simulink model "SISO_Timer"  (R2024a)
settings: Solver=VariableStepAuto  StartTime=0.0  StopTime=30  RelTol=1e-3
undefined symbols (not defined in the file or in its folder): BOOL, DINT, slplc
(part 2 of 3)

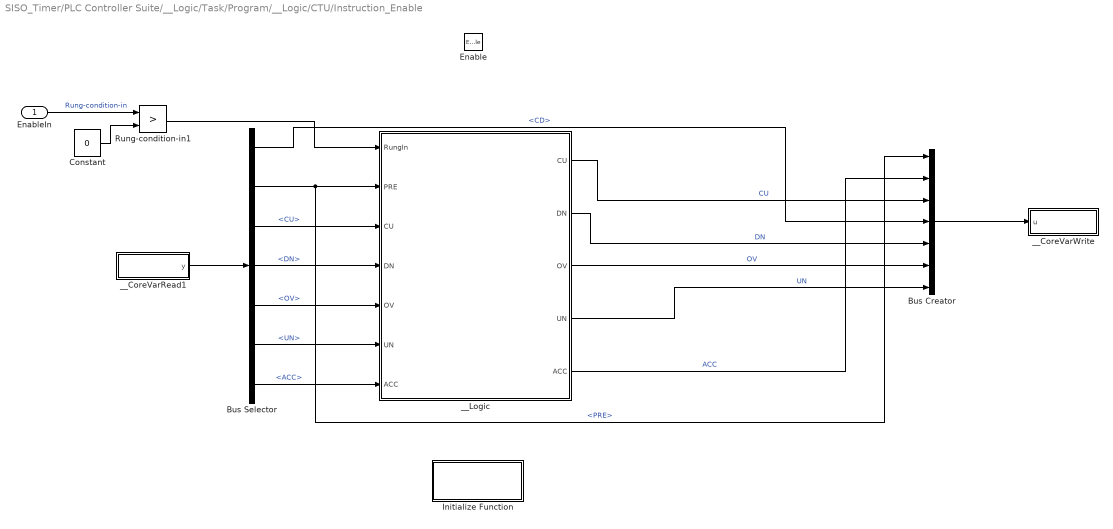
== system SISO_Timer/PLC Controller Suite/__Logic/Task/Program/__Logic/CTU/Instruction_Enable ==
  EnableIn : Inport
  Enable : EnablePort
  Bus Creator : BusCreator  Inputs=7  OutDataTypeStr=Bus: COUNTER  NonVirtualBus=on
  Bus Selector : BusSelector  OutputSignals=CD,PRE,CU,DN,OV,UN,ACC
  Constant : Constant  Value=0
  Initialize Function : Subsystem  TreatAsAtomicUnit=on
  Rung-condition-in1 : RelationalOperator  Operator=>  OutDataTypeStr=boolean  RndMeth=Simplest  InputSameDT=off
  __CoreVarRead1 : Subsystem  Tag=CoreVarReadBlock  DisableCoverage=on  TreatAsAtomicUnit=on  mask{PLCBlockType=CoreVarRead}
      mask init:
      | slplc.callbacks.initCoreVariable(gcb, 'read');
      mask Help: web([docroot '/plccoder/ref/__corevarread' '.html']);
      mask DialogControl PLCBlockTitle Prompt: Core Variable Read
  __CoreVarWrite : Subsystem  Tag=CoreVarWriteBlock  DisableCoverage=on  TreatAsAtomicUnit=on  mask{PLCBlockType=CoreVarWrite}
      mask init:
      | slplc.callbacks.initCoreVariable(gcb, 'write');
      mask Help: web([docroot '/plccoder/ref/__corevarwrite' '.html']);
      mask DialogControl PLCBlockTitle Prompt: Core Variable Write
  __Logic : MATLAB Function  Priority=12  DisableCoverage=on
  wires:
  Rung-condition-in1/1 -> __Logic/1(RungIn)
  Bus Selector/5 -> __Logic/5("OV ")  "<OV>"
  __Logic/4(UN) -> Bus Creator/7  "UN"
  Bus Selector/7 -> __Logic/7("ACC ")  "<ACC>"
  Bus Creator/1 -> __CoreVarWrite/1(u)
  __Logic/2(DN) -> Bus Creator/5  "DN"
  __Logic/1(CU) -> Bus Creator/3  "CU"
  __Logic/5(ACC) -> Bus Creator/2  "ACC"
  Bus Selector/6 -> __Logic/6("UN ")  "<UN>"
  __Logic/3(OV) -> Bus Creator/6  "OV"
  Bus Selector/2 -> __Logic/2(PRE), Bus Creator/1  "<PRE>"
  __CoreVarRead1/1(y) -> Bus Selector/1
  Bus Selector/3 -> __Logic/3("CU ")  "<CU>"
  Bus Selector/1 -> Bus Creator/4  "<CD>"
  Bus Selector/4 -> __Logic/4("DN ")  "<DN>"
  Constant/1 -> Rung-condition-in1/2
  EnableIn/1 -> Rung-condition-in1/1  "Rung-condition-in"

== system SISO_Timer/PLC Controller Suite/__Logic/Task/Program/__Logic/CTU/RungInOverride ==
  In1 : Inport
  AND : Logic  AllPortsSameDT=off  OutDataTypeStr=boolean
  ForceRungInFalseRead : Subsystem  DisableCoverage=on  TreatAsAtomicUnit=on  mask{PLCLabelTag=_Force_RungIn_False, PLCBlockType=ForceRungInFalseRead}
      mask prompts: PLCLabelTag "Label Tag:"
      mask init:
      | block = gcb;
      | maskObj = Simulink.Mask.get(block);
      | maskObj.Display = sprintf('disp(''%s'');', PLCLabelTag);
      mask Help: web([docroot '/plccoder/ref/forcerunginfalseread' '.html']);
      mask DialogControl PLCBlockTitle Prompt: Force Rung-In False Read
      mask Display: disp('_Force_RungIn_False');
  NOT : Logic  Operator=NOT  IconShape=distinctive  AllPortsSameDT=off  OutDataTypeStr=boolean
  Out1 : Outport  VectorParamsAs1DForOutWhenUnconnected=off
  wires:
  AND/1 -> Out1/1
  In1/1 -> AND/2
  ForceRungInFalseRead/1(Out1) -> NOT/1
  NOT/1 -> AND/1

== system SISO_Timer/PLC Controller Suite/__Logic/Task/Program/__Logic/CTU/__CoreVarRead ==
  DataRead : DataStoreRead  DataStoreName=xxx_PLC_VAR_T  IndexOptions=Index vector (dialog)  Indices=1  OutputSizes=1
  y : Outport  VectorParamsAs1DForOutWhenUnconnected=off
  wires:
  DataRead/1 -> y/1

== system SISO_Timer/PLC Controller Suite/__Logic/Task/Program/__Logic/Junction/BlockEnableRead ==
  __CoreLabelRead : Subsystem  Tag=CoreVarReadBlock  DisableCoverage=on  TreatAsAtomicUnit=on  mask{PLCBlockType=CoreLabelRead}
      mask init:
      | slplc.callbacks.initRoutineLabelRead(gcb);
      mask Help: web([docroot '/plccoder/ref/__corelabelread' '.html']);
      mask DialogControl PLCBlockTitle Prompt: Core Label Read
  Out1 : Outport  VectorParamsAs1DForOutWhenUnconnected=off
  wires:
  __CoreLabelRead/1(Out1) -> Out1/1

== system SISO_Timer/PLC Controller Suite/__Logic/Task/Program/__Logic/Junction/__Enable ==
  RungIn1 : Inport
  RungIn2 : Inport  Port=2
  Enable : EnablePort
  Logical Operator : Logic  Operator=OR  AllPortsSameDT=off  OutDataTypeStr=BOOL
  RungOut : Outport  VectorParamsAs1DForOutWhenUnconnected=off
  wires:
  RungIn2/1 -> Logical Operator/2
  Logical Operator/1 -> RungOut/1
  RungIn1/1 -> Logical Operator/1

== system SISO_Timer/PLC Controller Suite/__Logic/Task/Program/__Logic/Junction1/BlockEnableRead ==
  __CoreLabelRead : Subsystem  Tag=CoreVarReadBlock  DisableCoverage=on  TreatAsAtomicUnit=on  mask{PLCBlockType=CoreLabelRead}
      mask init:
      | slplc.callbacks.initRoutineLabelRead(gcb);
      mask Help: web([docroot '/plccoder/ref/__corelabelread' '.html']);
      mask DialogControl PLCBlockTitle Prompt: Core Label Read
  Out1 : Outport  VectorParamsAs1DForOutWhenUnconnected=off
  wires:
  __CoreLabelRead/1(Out1) -> Out1/1

== system SISO_Timer/PLC Controller Suite/__Logic/Task/Program/__Logic/Junction1/__Enable ==
  RungIn1 : Inport
  RungIn2 : Inport  Port=2
  Enable : EnablePort
  Logical Operator : Logic  Operator=OR  AllPortsSameDT=off  OutDataTypeStr=BOOL
  RungOut : Outport  VectorParamsAs1DForOutWhenUnconnected=off
  wires:
  RungIn2/1 -> Logical Operator/2
  Logical Operator/1 -> RungOut/1
  RungIn1/1 -> Logical Operator/1

== system SISO_Timer/PLC Controller Suite/__Logic/Task/Program/__Logic/OTE/BlockEnableRead ==
  __CoreLabelRead : Subsystem  Tag=CoreVarReadBlock  DisableCoverage=on  TreatAsAtomicUnit=on  mask{PLCBlockType=CoreLabelRead}
      mask init:
      | slplc.callbacks.initRoutineLabelRead(gcb);
      mask Help: web([docroot '/plccoder/ref/__corelabelread' '.html']);
      mask DialogControl PLCBlockTitle Prompt: Core Label Read
  Out1 : Outport  VectorParamsAs1DForOutWhenUnconnected=off
  wires:
  __CoreLabelRead/1(Out1) -> Out1/1

== system SISO_Timer/PLC Controller Suite/__Logic/Task/Program/__Logic/OTE/Instruction_Enable ==
  Rung-condition-in : Inport  OutDataTypeStr=BOOL
  Enable : EnablePort
  Initialize Function : Subsystem  TreatAsAtomicUnit=on
  NOT : Logic  Operator=NOT  IconShape=distinctive  AllPortsSameDT=off  OutDataTypeStr=boolean
  Rung-condition is false : Subsystem  Priority=12  DisableCoverage=on
  Rung-condition-in is true : Subsystem  Priority=12  DisableCoverage=on
  wires:
  NOT/1 -> Rung-condition is false/Enable
  Rung-condition-in/1 -> Rung-condition-in is true/Enable, NOT/1  "Rung-condition-in"

== system SISO_Timer/PLC Controller Suite/__Logic/Task/Program/__Logic/OTE/RungInOverride ==
  In1 : Inport
  AND : Logic  AllPortsSameDT=off  OutDataTypeStr=boolean
  ForceRungInFalseRead : Subsystem  DisableCoverage=on  TreatAsAtomicUnit=on  mask{PLCLabelTag=_Force_RungIn_False, PLCBlockType=ForceRungInFalseRead}
      mask prompts: PLCLabelTag "Label Tag:"
      mask init:
      | block = gcb;
      | maskObj = Simulink.Mask.get(block);
      | maskObj.Display = sprintf('disp(''%s'');', PLCLabelTag);
      mask Help: web([docroot '/plccoder/ref/forcerunginfalseread' '.html']);
      mask DialogControl PLCBlockTitle Prompt: Force Rung-In False Read
      mask Display: disp('_Force_RungIn_False');
  NOT : Logic  Operator=NOT  IconShape=distinctive  AllPortsSameDT=off  OutDataTypeStr=boolean
  Out1 : Outport  VectorParamsAs1DForOutWhenUnconnected=off
  wires:
  AND/1 -> Out1/1
  In1/1 -> AND/2
  ForceRungInFalseRead/1(Out1) -> NOT/1
  NOT/1 -> AND/1

== system SISO_Timer/PLC Controller Suite/__Logic/Task/Program/__Logic/OTE/__CoreVarRead ==
  DataRead : DataStoreRead  DataStoreName=xxx_PLC_VAR_St2  IndexOptions=Index vector (dialog)  Indices=1  OutputSizes=1
  y : Outport  VectorParamsAs1DForOutWhenUnconnected=off
  wires:
  DataRead/1 -> y/1

== system SISO_Timer/PLC Controller Suite/__Logic/Task/Program/__Logic/OTE1/BlockEnableRead ==
  __CoreLabelRead : Subsystem  Tag=CoreVarReadBlock  DisableCoverage=on  TreatAsAtomicUnit=on  mask{PLCBlockType=CoreLabelRead}
      mask init:
      | slplc.callbacks.initRoutineLabelRead(gcb);
      mask Help: web([docroot '/plccoder/ref/__corelabelread' '.html']);
      mask DialogControl PLCBlockTitle Prompt: Core Label Read
  Out1 : Outport  VectorParamsAs1DForOutWhenUnconnected=off
  wires:
  __CoreLabelRead/1(Out1) -> Out1/1

== system SISO_Timer/PLC Controller Suite/__Logic/Task/Program/__Logic/OTE1/Instruction_Enable ==
  Rung-condition-in : Inport  OutDataTypeStr=BOOL
  Enable : EnablePort
  Initialize Function : Subsystem  TreatAsAtomicUnit=on
  NOT : Logic  Operator=NOT  IconShape=distinctive  AllPortsSameDT=off  OutDataTypeStr=boolean
  Rung-condition is false : Subsystem  Priority=12  DisableCoverage=on
  Rung-condition-in is true : Subsystem  Priority=12  DisableCoverage=on
  wires:
  NOT/1 -> Rung-condition is false/Enable
  Rung-condition-in/1 -> Rung-condition-in is true/Enable, NOT/1  "Rung-condition-in"

== system SISO_Timer/PLC Controller Suite/__Logic/Task/Program/__Logic/OTE1/RungInOverride ==
  In1 : Inport
  AND : Logic  AllPortsSameDT=off  OutDataTypeStr=boolean
  ForceRungInFalseRead : Subsystem  DisableCoverage=on  TreatAsAtomicUnit=on  mask{PLCLabelTag=_Force_RungIn_False, PLCBlockType=ForceRungInFalseRead}
      mask prompts: PLCLabelTag "Label Tag:"
      mask init:
      | block = gcb;
      | maskObj = Simulink.Mask.get(block);
      | maskObj.Display = sprintf('disp(''%s'');', PLCLabelTag);
      mask Help: web([docroot '/plccoder/ref/forcerunginfalseread' '.html']);
      mask DialogControl PLCBlockTitle Prompt: Force Rung-In False Read
      mask Display: disp('_Force_RungIn_False');
  NOT : Logic  Operator=NOT  IconShape=distinctive  AllPortsSameDT=off  OutDataTypeStr=boolean
  Out1 : Outport  VectorParamsAs1DForOutWhenUnconnected=off
  wires:
  AND/1 -> Out1/1
  In1/1 -> AND/2
  ForceRungInFalseRead/1(Out1) -> NOT/1
  NOT/1 -> AND/1

== system SISO_Timer/PLC Controller Suite/__Logic/Task/Program/__Logic/OTE1/__CoreVarRead ==
  DataRead : DataStoreRead  DataStoreName=xxx_PLC_VAR_St1  IndexOptions=Index vector (dialog)  Indices=1  OutputSizes=1
  y : Outport  VectorParamsAs1DForOutWhenUnconnected=off
  wires:
  DataRead/1 -> y/1

== system SISO_Timer/PLC Controller Suite/__Logic/Task/Program/__Logic/OTE2/BlockEnableRead ==
  __CoreLabelRead : Subsystem  Tag=CoreVarReadBlock  DisableCoverage=on  TreatAsAtomicUnit=on  mask{PLCBlockType=CoreLabelRead}
      mask init:
      | slplc.callbacks.initRoutineLabelRead(gcb);
      mask Help: web([docroot '/plccoder/ref/__corelabelread' '.html']);
      mask DialogControl PLCBlockTitle Prompt: Core Label Read
  Out1 : Outport  VectorParamsAs1DForOutWhenUnconnected=off
  wires:
  __CoreLabelRead/1(Out1) -> Out1/1

== system SISO_Timer/PLC Controller Suite/__Logic/Task/Program/__Logic/OTE2/Instruction_Enable ==
  Rung-condition-in : Inport  OutDataTypeStr=BOOL
  Enable : EnablePort
  Initialize Function : Subsystem  TreatAsAtomicUnit=on
  NOT : Logic  Operator=NOT  IconShape=distinctive  AllPortsSameDT=off  OutDataTypeStr=boolean
  Rung-condition is false : Subsystem  Priority=12  DisableCoverage=on
  Rung-condition-in is true : Subsystem  Priority=12  DisableCoverage=on
  wires:
  NOT/1 -> Rung-condition is false/Enable
  Rung-condition-in/1 -> Rung-condition-in is true/Enable, NOT/1  "Rung-condition-in"

== system SISO_Timer/PLC Controller Suite/__Logic/Task/Program/__Logic/OTE2/RungInOverride ==
  In1 : Inport
  AND : Logic  AllPortsSameDT=off  OutDataTypeStr=boolean
  ForceRungInFalseRead : Subsystem  DisableCoverage=on  TreatAsAtomicUnit=on  mask{PLCLabelTag=_Force_RungIn_False, PLCBlockType=ForceRungInFalseRead}
      mask prompts: PLCLabelTag "Label Tag:"
      mask init:
      | block = gcb;
      | maskObj = Simulink.Mask.get(block);
      | maskObj.Display = sprintf('disp(''%s'');', PLCLabelTag);
      mask Help: web([docroot '/plccoder/ref/forcerunginfalseread' '.html']);
      mask DialogControl PLCBlockTitle Prompt: Force Rung-In False Read
      mask Display: disp('_Force_RungIn_False');
  NOT : Logic  Operator=NOT  IconShape=distinctive  AllPortsSameDT=off  OutDataTypeStr=boolean
  Out1 : Outport  VectorParamsAs1DForOutWhenUnconnected=off
  wires:
  AND/1 -> Out1/1
  In1/1 -> AND/2
  ForceRungInFalseRead/1(Out1) -> NOT/1
  NOT/1 -> AND/1

== system SISO_Timer/PLC Controller Suite/__Logic/Task/Program/__Logic/OTE2/__CoreVarRead ==
  DataRead : DataStoreRead  DataStoreName=xxx_PLC_VAR_Motor  IndexOptions=Index vector (dialog)  Indices=1  OutputSizes=1
  y : Outport  VectorParamsAs1DForOutWhenUnconnected=off
  wires:
  DataRead/1 -> y/1

== system SISO_Timer/PLC Controller Suite/__Logic/Task/Program/__Logic/XIC/BlockEnableRead ==
  __CoreLabelRead : Subsystem  Tag=CoreVarReadBlock  DisableCoverage=on  TreatAsAtomicUnit=on  mask{PLCBlockType=CoreLabelRead}
      mask init:
      | slplc.callbacks.initRoutineLabelRead(gcb);
      mask Help: web([docroot '/plccoder/ref/__corelabelread' '.html']);
      mask DialogControl PLCBlockTitle Prompt: Core Label Read
  Out1 : Outport  VectorParamsAs1DForOutWhenUnconnected=off
  wires:
  __CoreLabelRead/1(Out1) -> Out1/1

== system SISO_Timer/PLC Controller Suite/__Logic/Task/Program/__Logic/XIC/Instruction_Enable ==
  Rung-condition-in : Inport  OutDataTypeStr=BOOL
  Enable : EnablePort
  Logical Operator : Logic  OutDataTypeStr=BOOL
  __CoreVarRead : Subsystem  Tag=CoreVarReadBlock  DisableCoverage=on  TreatAsAtomicUnit=on  mask{PLCBlockType=CoreVarRead}
      mask init:
      | slplc.callbacks.initCoreVariable(gcb, 'read');
      mask Help: web([docroot '/plccoder/ref/__corevarread' '.html']);
      mask DialogControl PLCBlockTitle Prompt: Core Variable Read
  Rung-condition-out : Outport  VectorParamsAs1DForOutWhenUnconnected=off
  wires:
  Rung-condition-in/1 -> Logical Operator/1  "Rung-condition-in"
  Logical Operator/1 -> Rung-condition-out/1  "Rung-condition-out"
  __CoreVarRead/1(y) -> Logical Operator/2  "DataBit"

== system SISO_Timer/PLC Controller Suite/__Logic/Task/Program/__Logic/XIC/RungInOverride ==
  In1 : Inport
  AND : Logic  AllPortsSameDT=off  OutDataTypeStr=boolean
  ForceRungInFalseRead : Subsystem  DisableCoverage=on  TreatAsAtomicUnit=on  mask{PLCLabelTag=_Force_RungIn_False, PLCBlockType=ForceRungInFalseRead}
      mask prompts: PLCLabelTag "Label Tag:"
      mask init:
      | block = gcb;
      | maskObj = Simulink.Mask.get(block);
      | maskObj.Display = sprintf('disp(''%s'');', PLCLabelTag);
      mask Help: web([docroot '/plccoder/ref/forcerunginfalseread' '.html']);
      mask DialogControl PLCBlockTitle Prompt: Force Rung-In False Read
      mask Display: disp('_Force_RungIn_False');
  NOT : Logic  Operator=NOT  IconShape=distinctive  AllPortsSameDT=off  OutDataTypeStr=boolean
  Out1 : Outport  VectorParamsAs1DForOutWhenUnconnected=off
  wires:
  AND/1 -> Out1/1
  In1/1 -> AND/2
  ForceRungInFalseRead/1(Out1) -> NOT/1
  NOT/1 -> AND/1

== system SISO_Timer/PLC Controller Suite/__Logic/Task/Program/__Logic/XIC/__CoreVarRead ==
  DataRead : DataStoreRead  DataStoreName=xxx_PLC_VAR_St1  IndexOptions=Index vector (dialog)  Indices=1  OutputSizes=1
  y : Outport  VectorParamsAs1DForOutWhenUnconnected=off
  wires:
  DataRead/1 -> y/1

== system SISO_Timer/PLC Controller Suite/__Logic/Task/Program/__Logic/XIC1/BlockEnableRead ==
  __CoreLabelRead : Subsystem  Tag=CoreVarReadBlock  DisableCoverage=on  TreatAsAtomicUnit=on  mask{PLCBlockType=CoreLabelRead}
      mask init:
      | slplc.callbacks.initRoutineLabelRead(gcb);
      mask Help: web([docroot '/plccoder/ref/__corelabelread' '.html']);
      mask DialogControl PLCBlockTitle Prompt: Core Label Read
  Out1 : Outport  VectorParamsAs1DForOutWhenUnconnected=off
  wires:
  __CoreLabelRead/1(Out1) -> Out1/1

== system SISO_Timer/PLC Controller Suite/__Logic/Task/Program/__Logic/XIC1/Instruction_Enable ==
  Rung-condition-in : Inport  OutDataTypeStr=BOOL
  Enable : EnablePort
  Logical Operator : Logic  OutDataTypeStr=BOOL
  __CoreVarRead : Subsystem  Tag=CoreVarReadBlock  DisableCoverage=on  TreatAsAtomicUnit=on  mask{PLCBlockType=CoreVarRead}
      mask init:
      | slplc.callbacks.initCoreVariable(gcb, 'read');
      mask Help: web([docroot '/plccoder/ref/__corevarread' '.html']);
      mask DialogControl PLCBlockTitle Prompt: Core Variable Read
  Rung-condition-out : Outport  VectorParamsAs1DForOutWhenUnconnected=off
  wires:
  Rung-condition-in/1 -> Logical Operator/1  "Rung-condition-in"
  Logical Operator/1 -> Rung-condition-out/1  "Rung-condition-out"
  __CoreVarRead/1(y) -> Logical Operator/2  "DataBit"

== system SISO_Timer/PLC Controller Suite/__Logic/Task/Program/__Logic/XIC1/RungInOverride ==
  In1 : Inport
  AND : Logic  AllPortsSameDT=off  OutDataTypeStr=boolean
  ForceRungInFalseRead : Subsystem  DisableCoverage=on  TreatAsAtomicUnit=on  mask{PLCLabelTag=_Force_RungIn_False, PLCBlockType=ForceRungInFalseRead}
      mask prompts: PLCLabelTag "Label Tag:"
      mask init:
      | block = gcb;
      | maskObj = Simulink.Mask.get(block);
      | maskObj.Display = sprintf('disp(''%s'');', PLCLabelTag);
      mask Help: web([docroot '/plccoder/ref/forcerunginfalseread' '.html']);
      mask DialogControl PLCBlockTitle Prompt: Force Rung-In False Read
      mask Display: disp('_Force_RungIn_False');
  NOT : Logic  Operator=NOT  IconShape=distinctive  AllPortsSameDT=off  OutDataTypeStr=boolean
  Out1 : Outport  VectorParamsAs1DForOutWhenUnconnected=off
  wires:
  AND/1 -> Out1/1
  In1/1 -> AND/2
  ForceRungInFalseRead/1(Out1) -> NOT/1
  NOT/1 -> AND/1

== system SISO_Timer/PLC Controller Suite/__Logic/Task/Program/__Logic/XIC1/__CoreVarRead ==
  DataRead : DataStoreRead  DataStoreName=xxx_PLC_VAR_Button  IndexOptions=Index vector (dialog)  Indices=1  OutputSizes=1
  y : Outport  VectorParamsAs1DForOutWhenUnconnected=off
  wires:
  DataRead/1 -> y/1

== system SISO_Timer/PLC Controller Suite/__Logic/Task/Program/__Logic/XIC2/BlockEnableRead ==
  __CoreLabelRead : Subsystem  Tag=CoreVarReadBlock  DisableCoverage=on  TreatAsAtomicUnit=on  mask{PLCBlockType=CoreLabelRead}
      mask init:
      | slplc.callbacks.initRoutineLabelRead(gcb);
      mask Help: web([docroot '/plccoder/ref/__corelabelread' '.html']);
      mask DialogControl PLCBlockTitle Prompt: Core Label Read
  Out1 : Outport  VectorParamsAs1DForOutWhenUnconnected=off
  wires:
  __CoreLabelRead/1(Out1) -> Out1/1

== system SISO_Timer/PLC Controller Suite/__Logic/Task/Program/__Logic/XIC2/Instruction_Enable ==
  Rung-condition-in : Inport  OutDataTypeStr=BOOL
  Enable : EnablePort
  Logical Operator : Logic  OutDataTypeStr=BOOL
  __CoreVarRead : Subsystem  Tag=CoreVarReadBlock  DisableCoverage=on  TreatAsAtomicUnit=on  mask{PLCBlockType=CoreVarRead}
      mask init:
      | slplc.callbacks.initCoreVariable(gcb, 'read');
      mask Help: web([docroot '/plccoder/ref/__corevarread' '.html']);
      mask DialogControl PLCBlockTitle Prompt: Core Variable Read
  Rung-condition-out : Outport  VectorParamsAs1DForOutWhenUnconnected=off
  wires:
  Rung-condition-in/1 -> Logical Operator/1  "Rung-condition-in"
  Logical Operator/1 -> Rung-condition-out/1  "Rung-condition-out"
  __CoreVarRead/1(y) -> Logical Operator/2  "DataBit"

== system SISO_Timer/PLC Controller Suite/__Logic/Task/Program/__Logic/XIC2/RungInOverride ==
  In1 : Inport
  AND : Logic  AllPortsSameDT=off  OutDataTypeStr=boolean
  ForceRungInFalseRead : Subsystem  DisableCoverage=on  TreatAsAtomicUnit=on  mask{PLCLabelTag=_Force_RungIn_False, PLCBlockType=ForceRungInFalseRead}
      mask prompts: PLCLabelTag "Label Tag:"
      mask init:
      | block = gcb;
      | maskObj = Simulink.Mask.get(block);
      | maskObj.Display = sprintf('disp(''%s'');', PLCLabelTag);
      mask Help: web([docroot '/plccoder/ref/forcerunginfalseread' '.html']);
      mask DialogControl PLCBlockTitle Prompt: Force Rung-In False Read
      mask Display: disp('_Force_RungIn_False');
  NOT : Logic  Operator=NOT  IconShape=distinctive  AllPortsSameDT=off  OutDataTypeStr=boolean
  Out1 : Outport  VectorParamsAs1DForOutWhenUnconnected=off
  wires:
  AND/1 -> Out1/1
  In1/1 -> AND/2
  ForceRungInFalseRead/1(Out1) -> NOT/1
  NOT/1 -> AND/1

== system SISO_Timer/PLC Controller Suite/__Logic/Task/Program/__Logic/XIC2/__CoreVarRead ==
  DataRead : DataStoreRead  DataStoreName=xxx_PLC_VAR_St2  IndexOptions=Index vector (dialog)  Indices=1  OutputSizes=1
  y : Outport  VectorParamsAs1DForOutWhenUnconnected=off
  wires:
  DataRead/1 -> y/1

== system SISO_Timer/PLC Controller Suite/__Logic/Task/Program/__Logic/XIC3/BlockEnableRead ==
  __CoreLabelRead : Subsystem  Tag=CoreVarReadBlock  DisableCoverage=on  TreatAsAtomicUnit=on  mask{PLCBlockType=CoreLabelRead}
      mask init:
      | slplc.callbacks.initRoutineLabelRead(gcb);
      mask Help: web([docroot '/plccoder/ref/__corelabelread' '.html']);
      mask DialogControl PLCBlockTitle Prompt: Core Label Read
  Out1 : Outport  VectorParamsAs1DForOutWhenUnconnected=off
  wires:
  __CoreLabelRead/1(Out1) -> Out1/1

== system SISO_Timer/PLC Controller Suite/__Logic/Task/Program/__Logic/XIC3/Instruction_Enable ==
  Rung-condition-in : Inport  OutDataTypeStr=BOOL
  Enable : EnablePort
  Logical Operator : Logic  OutDataTypeStr=BOOL
  __CoreVarRead : Subsystem  Tag=CoreVarReadBlock  DisableCoverage=on  TreatAsAtomicUnit=on  mask{PLCBlockType=CoreVarRead}
      mask init:
      | slplc.callbacks.initCoreVariable(gcb, 'read');
      mask Help: web([docroot '/plccoder/ref/__corevarread' '.html']);
      mask DialogControl PLCBlockTitle Prompt: Core Variable Read
  Rung-condition-out : Outport  VectorParamsAs1DForOutWhenUnconnected=off
  wires:
  Rung-condition-in/1 -> Logical Operator/1  "Rung-condition-in"
  Logical Operator/1 -> Rung-condition-out/1  "Rung-condition-out"
  __CoreVarRead/1(y) -> Logical Operator/2  "DataBit"

== system SISO_Timer/PLC Controller Suite/__Logic/Task/Program/__Logic/XIC3/RungInOverride ==
  In1 : Inport
  AND : Logic  AllPortsSameDT=off  OutDataTypeStr=boolean
  ForceRungInFalseRead : Subsystem  DisableCoverage=on  TreatAsAtomicUnit=on  mask{PLCLabelTag=_Force_RungIn_False, PLCBlockType=ForceRungInFalseRead}
      mask prompts: PLCLabelTag "Label Tag:"
      mask init:
      | block = gcb;
      | maskObj = Simulink.Mask.get(block);
      | maskObj.Display = sprintf('disp(''%s'');', PLCLabelTag);
      mask Help: web([docroot '/plccoder/ref/forcerunginfalseread' '.html']);
      mask DialogControl PLCBlockTitle Prompt: Force Rung-In False Read
      mask Display: disp('_Force_RungIn_False');
  NOT : Logic  Operator=NOT  IconShape=distinctive  AllPortsSameDT=off  OutDataTypeStr=boolean
  Out1 : Outport  VectorParamsAs1DForOutWhenUnconnected=off
  wires:
  AND/1 -> Out1/1
  In1/1 -> AND/2
  ForceRungInFalseRead/1(Out1) -> NOT/1
  NOT/1 -> AND/1

== system SISO_Timer/PLC Controller Suite/__Logic/Task/Program/__Logic/XIC3/__CoreVarRead ==
  DataRead : DataStoreRead  DataStoreName=xxx_PLC_VAR_T  DataStoreElements=xxx_PLC_VAR_T.DN  IndexOptions=Index vector (dialog)  Indices=1  OutputSizes=1
  y : Outport  VectorParamsAs1DForOutWhenUnconnected=off
  wires:
  DataRead/1 -> y/1

== system SISO_Timer/PLC Controller Suite/__Logic/Task/Program/__Logic/XIC4/BlockEnableRead ==
  __CoreLabelRead : Subsystem  Tag=CoreVarReadBlock  DisableCoverage=on  TreatAsAtomicUnit=on  mask{PLCBlockType=CoreLabelRead}
      mask init:
      | slplc.callbacks.initRoutineLabelRead(gcb);
      mask Help: web([docroot '/plccoder/ref/__corelabelread' '.html']);
      mask DialogControl PLCBlockTitle Prompt: Core Label Read
  Out1 : Outport  VectorParamsAs1DForOutWhenUnconnected=off
  wires:
  __CoreLabelRead/1(Out1) -> Out1/1

== system SISO_Timer/PLC Controller Suite/__Logic/Task/Program/__Logic/XIC4/Instruction_Enable ==
  Rung-condition-in : Inport  OutDataTypeStr=BOOL
  Enable : EnablePort
  Logical Operator : Logic  OutDataTypeStr=BOOL
  __CoreVarRead : Subsystem  Tag=CoreVarReadBlock  DisableCoverage=on  TreatAsAtomicUnit=on  mask{PLCBlockType=CoreVarRead}
      mask init:
      | slplc.callbacks.initCoreVariable(gcb, 'read');
      mask Help: web([docroot '/plccoder/ref/__corevarread' '.html']);
      mask DialogControl PLCBlockTitle Prompt: Core Variable Read
  Rung-condition-out : Outport  VectorParamsAs1DForOutWhenUnconnected=off
  wires:
  Rung-condition-in/1 -> Logical Operator/1  "Rung-condition-in"
  Logical Operator/1 -> Rung-condition-out/1  "Rung-condition-out"
  __CoreVarRead/1(y) -> Logical Operator/2  "DataBit"

== system SISO_Timer/PLC Controller Suite/__Logic/Task/Program/__Logic/XIC4/RungInOverride ==
  In1 : Inport
  AND : Logic  AllPortsSameDT=off  OutDataTypeStr=boolean
  ForceRungInFalseRead : Subsystem  DisableCoverage=on  TreatAsAtomicUnit=on  mask{PLCLabelTag=_Force_RungIn_False, PLCBlockType=ForceRungInFalseRead}
      mask prompts: PLCLabelTag "Label Tag:"
      mask init:
      | block = gcb;
      | maskObj = Simulink.Mask.get(block);
      | maskObj.Display = sprintf('disp(''%s'');', PLCLabelTag);
      mask Help: web([docroot '/plccoder/ref/forcerunginfalseread' '.html']);
      mask DialogControl PLCBlockTitle Prompt: Force Rung-In False Read
      mask Display: disp('_Force_RungIn_False');
  NOT : Logic  Operator=NOT  IconShape=distinctive  AllPortsSameDT=off  OutDataTypeStr=boolean
  Out1 : Outport  VectorParamsAs1DForOutWhenUnconnected=off
  wires:
  AND/1 -> Out1/1
  In1/1 -> AND/2
  ForceRungInFalseRead/1(Out1) -> NOT/1
  NOT/1 -> AND/1

== system SISO_Timer/PLC Controller Suite/__Logic/Task/Program/__Logic/XIC4/__CoreVarRead ==
  DataRead : DataStoreRead  DataStoreName=xxx_PLC_VAR_St2  IndexOptions=Index vector (dialog)  Indices=1  OutputSizes=1
  y : Outport  VectorParamsAs1DForOutWhenUnconnected=off
  wires:
  DataRead/1 -> y/1

== system SISO_Timer/PLC Controller Suite/__Logic/Task/Program/__Logic/XIC5/BlockEnableRead ==
  __CoreLabelRead : Subsystem  Tag=CoreVarReadBlock  DisableCoverage=on  TreatAsAtomicUnit=on  mask{PLCBlockType=CoreLabelRead}
      mask init:
      | slplc.callbacks.initRoutineLabelRead(gcb);
      mask Help: web([docroot '/plccoder/ref/__corelabelread' '.html']);
      mask DialogControl PLCBlockTitle Prompt: Core Label Read
  Out1 : Outport  VectorParamsAs1DForOutWhenUnconnected=off
  wires:
  __CoreLabelRead/1(Out1) -> Out1/1

== system SISO_Timer/PLC Controller Suite/__Logic/Task/Program/__Logic/XIC5/Instruction_Enable ==
  Rung-condition-in : Inport  OutDataTypeStr=BOOL
  Enable : EnablePort
  Logical Operator : Logic  OutDataTypeStr=BOOL
  __CoreVarRead : Subsystem  Tag=CoreVarReadBlock  DisableCoverage=on  TreatAsAtomicUnit=on  mask{PLCBlockType=CoreVarRead}
      mask init:
      | slplc.callbacks.initCoreVariable(gcb, 'read');
      mask Help: web([docroot '/plccoder/ref/__corevarread' '.html']);
      mask DialogControl PLCBlockTitle Prompt: Core Variable Read
  Rung-condition-out : Outport  VectorParamsAs1DForOutWhenUnconnected=off
  wires:
  Rung-condition-in/1 -> Logical Operator/1  "Rung-condition-in"
  Logical Operator/1 -> Rung-condition-out/1  "Rung-condition-out"
  __CoreVarRead/1(y) -> Logical Operator/2  "DataBit"

== system SISO_Timer/PLC Controller Suite/__Logic/Task/Program/__Logic/XIC5/RungInOverride ==
  In1 : Inport
  AND : Logic  AllPortsSameDT=off  OutDataTypeStr=boolean
  ForceRungInFalseRead : Subsystem  DisableCoverage=on  TreatAsAtomicUnit=on  mask{PLCLabelTag=_Force_RungIn_False, PLCBlockType=ForceRungInFalseRead}
      mask prompts: PLCLabelTag "Label Tag:"
      mask init:
      | block = gcb;
      | maskObj = Simulink.Mask.get(block);
      | maskObj.Display = sprintf('disp(''%s'');', PLCLabelTag);
      mask Help: web([docroot '/plccoder/ref/forcerunginfalseread' '.html']);
      mask DialogControl PLCBlockTitle Prompt: Force Rung-In False Read
      mask Display: disp('_Force_RungIn_False');
  NOT : Logic  Operator=NOT  IconShape=distinctive  AllPortsSameDT=off  OutDataTypeStr=boolean
  Out1 : Outport  VectorParamsAs1DForOutWhenUnconnected=off
  wires:
  AND/1 -> Out1/1
  In1/1 -> AND/2
  ForceRungInFalseRead/1(Out1) -> NOT/1
  NOT/1 -> AND/1

== system SISO_Timer/PLC Controller Suite/__Logic/Task/Program/__Logic/XIC5/__CoreVarRead ==
  DataRead : DataStoreRead  DataStoreName=xxx_PLC_VAR_St2  IndexOptions=Index vector (dialog)  Indices=1  OutputSizes=1
  y : Outport  VectorParamsAs1DForOutWhenUnconnected=off
  wires:
  DataRead/1 -> y/1

== system SISO_Timer/PLC Controller Suite/__Logic/Task/Program/__Logic/XIO1/BlockEnableRead ==
  __CoreLabelRead : Subsystem  Tag=CoreVarReadBlock  DisableCoverage=on  TreatAsAtomicUnit=on  mask{PLCBlockType=CoreLabelRead}
      mask init:
      | slplc.callbacks.initRoutineLabelRead(gcb);
      mask Help: web([docroot '/plccoder/ref/__corelabelread' '.html']);
      mask DialogControl PLCBlockTitle Prompt: Core Label Read
  Out1 : Outport  VectorParamsAs1DForOutWhenUnconnected=off
  wires:
  __CoreLabelRead/1(Out1) -> Out1/1

== system SISO_Timer/PLC Controller Suite/__Logic/Task/Program/__Logic/XIO1/Instruction_Enable ==
  Rung-condition-in : Inport  OutDataTypeStr=BOOL
  Enable : EnablePort
  Logical Operator : Logic  OutDataTypeStr=BOOL
  NOT : Logic  DisableCoverage=on  Operator=NOT  IconShape=distinctive  OutDataTypeStr=BOOL
  __CoreVarRead : Subsystem  Tag=CoreVarReadBlock  DisableCoverage=on  TreatAsAtomicUnit=on  mask{PLCBlockType=CoreVarRead}
      mask init:
      | slplc.callbacks.initCoreVariable(gcb, 'read');
      mask Help: web([docroot '/plccoder/ref/__corevarread' '.html']);
      mask DialogControl PLCBlockTitle Prompt: Core Variable Read
  Rung-condition-out : Outport  VectorParamsAs1DForOutWhenUnconnected=off
  wires:
  Rung-condition-in/1 -> Logical Operator/1  "Rung-condition-in"
  Logical Operator/1 -> Rung-condition-out/1  "Rung-condition-out"
  __CoreVarRead/1(y) -> NOT/1  "DataBit"
  NOT/1 -> Logical Operator/2  "~DataBit"

== system SISO_Timer/PLC Controller Suite/__Logic/Task/Program/__Logic/XIO1/RungInOverride ==
  In1 : Inport
  AND : Logic  AllPortsSameDT=off  OutDataTypeStr=boolean
  ForceRungInFalseRead : Subsystem  DisableCoverage=on  TreatAsAtomicUnit=on  mask{PLCLabelTag=_Force_RungIn_False, PLCBlockType=ForceRungInFalseRead}
      mask prompts: PLCLabelTag "Label Tag:"
      mask init:
      | block = gcb;
      | maskObj = Simulink.Mask.get(block);
      | maskObj.Display = sprintf('disp(''%s'');', PLCLabelTag);
      mask Help: web([docroot '/plccoder/ref/forcerunginfalseread' '.html']);
      mask DialogControl PLCBlockTitle Prompt: Force Rung-In False Read
      mask Display: disp('_Force_RungIn_False');
  NOT : Logic  Operator=NOT  IconShape=distinctive  AllPortsSameDT=off  OutDataTypeStr=boolean
  Out1 : Outport  VectorParamsAs1DForOutWhenUnconnected=off
  wires:
  AND/1 -> Out1/1
  In1/1 -> AND/2
  ForceRungInFalseRead/1(Out1) -> NOT/1
  NOT/1 -> AND/1

== system SISO_Timer/PLC Controller Suite/__Logic/Task/Program/__Logic/XIO1/__CoreVarRead ==
  DataRead : DataStoreRead  DataStoreName=xxx_PLC_VAR_St2  IndexOptions=Index vector (dialog)  Indices=1  OutputSizes=1
  y : Outport  VectorParamsAs1DForOutWhenUnconnected=off
  wires:
  DataRead/1 -> y/1

== system SISO_Timer/PLC Controller Suite/__Logic/Task/Program/__Logic/CTU/BlockEnableRead/__CoreLabelRead ==
  DataRead : DataStoreRead  DataStoreName=x_PLCLabel__s4_3653__Block_Enable  IndexOptions=Index vector (dialog)  Indices=1  OutputSizes=1
  Out1 : Outport  VectorParamsAs1DForOutWhenUnconnected=off
  wires:
  DataRead/1 -> Out1/1

== system SISO_Timer/PLC Controller Suite/__Logic/Task/Program/__Logic/CTU/Instruction_Enable/Initialize Function ==
  Constant : Constant  OutDataTypeStr=BOOL
  Event Listener : EventListener  DisableCoverage=on  EventName=reset
  VarWrite1 : Subsystem  DisableCoverage=on  TreatAsAtomicUnit=on  mask{PLCOperandTag=CU, PLCOperandExpression=xxx_PLC_VAR_T.CU, PLCBlockType=VarWrite, PLCPOUType=VarWrite}
      mask prompts: PLCOperandTag "Operand Tag:"
      mask init:
      | slplc.callbacks.initInstruction(gcb);
      mask Help: web([docroot '/plccoder/ref/varwrite' '.html']);
      mask DialogControl PLCBlockTitle Prompt: Variable Write
      mask Display: disp(get_param(gcb, 'PLCOperandTag'));
  wires:
  Constant/1 -> VarWrite1/1(In1)

== system SISO_Timer/PLC Controller Suite/__Logic/Task/Program/__Logic/CTU/Instruction_Enable/__CoreVarRead1 ==
  DataRead : DataStoreRead  DataStoreName=xxx_PLC_VAR_T  IndexOptions=Index vector (dialog)  Indices=1  OutputSizes=1
  y : Outport  VectorParamsAs1DForOutWhenUnconnected=off
  wires:
  DataRead/1 -> y/1

== system SISO_Timer/PLC Controller Suite/__Logic/Task/Program/__Logic/CTU/Instruction_Enable/__CoreVarWrite ==
  u : Inport
  DataWrite : DataStoreWrite  DataStoreName=xxx_PLC_VAR_T  IndexOptions=Index vector (dialog)  Indices=1  OutputSizes=1
  wires:
  u/1 -> DataWrite/1

== system SISO_Timer/PLC Controller Suite/__Logic/Task/Program/__Logic/CTU/RungInOverride/ForceRungInFalseRead ==
  __CoreLabelRead : Subsystem  Tag=CoreVarReadBlock  DisableCoverage=on  TreatAsAtomicUnit=on  mask{PLCBlockType=CoreLabelRead}
      mask init:
      | slplc.callbacks.initRoutineLabelRead(gcb);
      mask Help: web([docroot '/plccoder/ref/__corelabelread' '.html']);
      mask DialogControl PLCBlockTitle Prompt: Core Label Read
  Out1 : Outport  VectorParamsAs1DForOutWhenUnconnected=off
  wires:
  __CoreLabelRead/1(Out1) -> Out1/1

== system SISO_Timer/PLC Controller Suite/__Logic/Task/Program/__Logic/Junction/BlockEnableRead/__CoreLabelRead ==
  DataRead : DataStoreRead  DataStoreName=x_PLCLabel__s4_3653__Block_Enable  IndexOptions=Index vector (dialog)  Indices=1  OutputSizes=1
  Out1 : Outport  VectorParamsAs1DForOutWhenUnconnected=off
  wires:
  DataRead/1 -> Out1/1

== system SISO_Timer/PLC Controller Suite/__Logic/Task/Program/__Logic/Junction1/BlockEnableRead/__CoreLabelRead ==
  DataRead : DataStoreRead  DataStoreName=x_PLCLabel__s4_3653__Block_Enable  IndexOptions=Index vector (dialog)  Indices=1  OutputSizes=1
  Out1 : Outport  VectorParamsAs1DForOutWhenUnconnected=off
  wires:
  DataRead/1 -> Out1/1

== system SISO_Timer/PLC Controller Suite/__Logic/Task/Program/__Logic/OTE/BlockEnableRead/__CoreLabelRead ==
  DataRead : DataStoreRead  DataStoreName=x_PLCLabel__s4_3653__Block_Enable  IndexOptions=Index vector (dialog)  Indices=1  OutputSizes=1
  Out1 : Outport  VectorParamsAs1DForOutWhenUnconnected=off
  wires:
  DataRead/1 -> Out1/1

== system SISO_Timer/PLC Controller Suite/__Logic/Task/Program/__Logic/OTE/Instruction_Enable/Initialize Function ==
  Constant : Constant  Value=0  OutDataTypeStr=BOOL
  Event Listener : EventListener  DisableCoverage=on  EventName=reset
  __CoreVarWrite : Subsystem  Tag=CoreVarWriteBlock  DisableCoverage=on  TreatAsAtomicUnit=on  mask{PLCBlockType=CoreVarWrite}
      mask init:
      | slplc.callbacks.initCoreVariable(gcb, 'write');
      mask Help: web([docroot '/plccoder/ref/__corevarwrite' '.html']);
      mask DialogControl PLCBlockTitle Prompt: Core Variable Write
  wires:
  Constant/1 -> __CoreVarWrite/1(u)

== system SISO_Timer/PLC Controller Suite/__Logic/Task/Program/__Logic/OTE/Instruction_Enable/Rung-condition is false ==
  Enable : EnablePort
  Constant : Constant  Value=0  OutDataTypeStr=BOOL
  __CoreVarWrite : Subsystem  Tag=CoreVarWriteBlock  DisableCoverage=on  TreatAsAtomicUnit=on  mask{PLCBlockType=CoreVarWrite}
      mask init:
      | slplc.callbacks.initCoreVariable(gcb, 'write');
      mask Help: web([docroot '/plccoder/ref/__corevarwrite' '.html']);
      mask DialogControl PLCBlockTitle Prompt: Core Variable Write
  wires:
  Constant/1 -> __CoreVarWrite/1(u)

== system SISO_Timer/PLC Controller Suite/__Logic/Task/Program/__Logic/OTE/Instruction_Enable/Rung-condition-in is true ==
  Enable : EnablePort
  Constant : Constant  OutDataTypeStr=BOOL
  __CoreVarWrite : Subsystem  Tag=CoreVarWriteBlock  DisableCoverage=on  TreatAsAtomicUnit=on  mask{PLCBlockType=CoreVarWrite}
      mask init:
      | slplc.callbacks.initCoreVariable(gcb, 'write');
      mask Help: web([docroot '/plccoder/ref/__corevarwrite' '.html']);
      mask DialogControl PLCBlockTitle Prompt: Core Variable Write
  wires:
  Constant/1 -> __CoreVarWrite/1(u)

== system SISO_Timer/PLC Controller Suite/__Logic/Task/Program/__Logic/OTE/RungInOverride/ForceRungInFalseRead ==
  __CoreLabelRead : Subsystem  Tag=CoreVarReadBlock  DisableCoverage=on  TreatAsAtomicUnit=on  mask{PLCBlockType=CoreLabelRead}
      mask init:
      | slplc.callbacks.initRoutineLabelRead(gcb);
      mask Help: web([docroot '/plccoder/ref/__corelabelread' '.html']);
      mask DialogControl PLCBlockTitle Prompt: Core Label Read
  Out1 : Outport  VectorParamsAs1DForOutWhenUnconnected=off
  wires:
  __CoreLabelRead/1(Out1) -> Out1/1

== system SISO_Timer/PLC Controller Suite/__Logic/Task/Program/__Logic/OTE1/BlockEnableRead/__CoreLabelRead ==
  DataRead : DataStoreRead  DataStoreName=x_PLCLabel__s4_3653__Block_Enable  IndexOptions=Index vector (dialog)  Indices=1  OutputSizes=1
  Out1 : Outport  VectorParamsAs1DForOutWhenUnconnected=off
  wires:
  DataRead/1 -> Out1/1

== system SISO_Timer/PLC Controller Suite/__Logic/Task/Program/__Logic/OTE1/Instruction_Enable/Initialize Function ==
  Constant : Constant  Value=0  OutDataTypeStr=BOOL
  Event Listener : EventListener  DisableCoverage=on  EventName=reset
  __CoreVarWrite : Subsystem  Tag=CoreVarWriteBlock  DisableCoverage=on  TreatAsAtomicUnit=on  mask{PLCBlockType=CoreVarWrite}
      mask init:
      | slplc.callbacks.initCoreVariable(gcb, 'write');
      mask Help: web([docroot '/plccoder/ref/__corevarwrite' '.html']);
      mask DialogControl PLCBlockTitle Prompt: Core Variable Write
  wires:
  Constant/1 -> __CoreVarWrite/1(u)

== system SISO_Timer/PLC Controller Suite/__Logic/Task/Program/__Logic/OTE1/Instruction_Enable/Rung-condition is false ==
  Enable : EnablePort
  Constant : Constant  Value=0  OutDataTypeStr=BOOL
  __CoreVarWrite : Subsystem  Tag=CoreVarWriteBlock  DisableCoverage=on  TreatAsAtomicUnit=on  mask{PLCBlockType=CoreVarWrite}
      mask init:
      | slplc.callbacks.initCoreVariable(gcb, 'write');
      mask Help: web([docroot '/plccoder/ref/__corevarwrite' '.html']);
      mask DialogControl PLCBlockTitle Prompt: Core Variable Write
  wires:
  Constant/1 -> __CoreVarWrite/1(u)

== system SISO_Timer/PLC Controller Suite/__Logic/Task/Program/__Logic/OTE1/Instruction_Enable/Rung-condition-in is true ==
  Enable : EnablePort
  Constant : Constant  OutDataTypeStr=BOOL
  __CoreVarWrite : Subsystem  Tag=CoreVarWriteBlock  DisableCoverage=on  TreatAsAtomicUnit=on  mask{PLCBlockType=CoreVarWrite}
      mask init:
      | slplc.callbacks.initCoreVariable(gcb, 'write');
      mask Help: web([docroot '/plccoder/ref/__corevarwrite' '.html']);
      mask DialogControl PLCBlockTitle Prompt: Core Variable Write
  wires:
  Constant/1 -> __CoreVarWrite/1(u)

== system SISO_Timer/PLC Controller Suite/__Logic/Task/Program/__Logic/OTE1/RungInOverride/ForceRungInFalseRead ==
  __CoreLabelRead : Subsystem  Tag=CoreVarReadBlock  DisableCoverage=on  TreatAsAtomicUnit=on  mask{PLCBlockType=CoreLabelRead}
      mask init:
      | slplc.callbacks.initRoutineLabelRead(gcb);
      mask Help: web([docroot '/plccoder/ref/__corelabelread' '.html']);
      mask DialogControl PLCBlockTitle Prompt: Core Label Read
  Out1 : Outport  VectorParamsAs1DForOutWhenUnconnected=off
  wires:
  __CoreLabelRead/1(Out1) -> Out1/1

== system SISO_Timer/PLC Controller Suite/__Logic/Task/Program/__Logic/OTE2/BlockEnableRead/__CoreLabelRead ==
  DataRead : DataStoreRead  DataStoreName=x_PLCLabel__s4_3653__Block_Enable  IndexOptions=Index vector (dialog)  Indices=1  OutputSizes=1
  Out1 : Outport  VectorParamsAs1DForOutWhenUnconnected=off
  wires:
  DataRead/1 -> Out1/1

== system SISO_Timer/PLC Controller Suite/__Logic/Task/Program/__Logic/OTE2/Instruction_Enable/Initialize Function ==
  Constant : Constant  Value=0  OutDataTypeStr=BOOL
  Event Listener : EventListener  DisableCoverage=on  EventName=reset
  __CoreVarWrite : Subsystem  Tag=CoreVarWriteBlock  DisableCoverage=on  TreatAsAtomicUnit=on  mask{PLCBlockType=CoreVarWrite}
      mask init:
      | slplc.callbacks.initCoreVariable(gcb, 'write');
      mask Help: web([docroot '/plccoder/ref/__corevarwrite' '.html']);
      mask DialogControl PLCBlockTitle Prompt: Core Variable Write
  wires:
  Constant/1 -> __CoreVarWrite/1(u)

== system SISO_Timer/PLC Controller Suite/__Logic/Task/Program/__Logic/OTE2/Instruction_Enable/Rung-condition is false ==
  Enable : EnablePort
  Constant : Constant  Value=0  OutDataTypeStr=BOOL
  __CoreVarWrite : Subsystem  Tag=CoreVarWriteBlock  DisableCoverage=on  TreatAsAtomicUnit=on  mask{PLCBlockType=CoreVarWrite}
      mask init:
      | slplc.callbacks.initCoreVariable(gcb, 'write');
      mask Help: web([docroot '/plccoder/ref/__corevarwrite' '.html']);
      mask DialogControl PLCBlockTitle Prompt: Core Variable Write
  wires:
  Constant/1 -> __CoreVarWrite/1(u)

== system SISO_Timer/PLC Controller Suite/__Logic/Task/Program/__Logic/OTE2/Instruction_Enable/Rung-condition-in is true ==
  Enable : EnablePort
  Constant : Constant  OutDataTypeStr=BOOL
  __CoreVarWrite : Subsystem  Tag=CoreVarWriteBlock  DisableCoverage=on  TreatAsAtomicUnit=on  mask{PLCBlockType=CoreVarWrite}
      mask init:
      | slplc.callbacks.initCoreVariable(gcb, 'write');
      mask Help: web([docroot '/plccoder/ref/__corevarwrite' '.html']);
      mask DialogControl PLCBlockTitle Prompt: Core Variable Write
  wires:
  Constant/1 -> __CoreVarWrite/1(u)

== system SISO_Timer/PLC Controller Suite/__Logic/Task/Program/__Logic/OTE2/RungInOverride/ForceRungInFalseRead ==
  __CoreLabelRead : Subsystem  Tag=CoreVarReadBlock  DisableCoverage=on  TreatAsAtomicUnit=on  mask{PLCBlockType=CoreLabelRead}
      mask init:
      | slplc.callbacks.initRoutineLabelRead(gcb);
      mask Help: web([docroot '/plccoder/ref/__corelabelread' '.html']);
      mask DialogControl PLCBlockTitle Prompt: Core Label Read
  Out1 : Outport  VectorParamsAs1DForOutWhenUnconnected=off
  wires:
  __CoreLabelRead/1(Out1) -> Out1/1

== system SISO_Timer/PLC Controller Suite/__Logic/Task/Program/__Logic/XIC/BlockEnableRead/__CoreLabelRead ==
  DataRead : DataStoreRead  DataStoreName=x_PLCLabel__s4_3653__Block_Enable  IndexOptions=Index vector (dialog)  Indices=1  OutputSizes=1
  Out1 : Outport  VectorParamsAs1DForOutWhenUnconnected=off
  wires:
  DataRead/1 -> Out1/1

== system SISO_Timer/PLC Controller Suite/__Logic/Task/Program/__Logic/XIC/Instruction_Enable/__CoreVarRead ==
  DataRead : DataStoreRead  DataStoreName=xxx_PLC_VAR_St1  IndexOptions=Index vector (dialog)  Indices=1  OutputSizes=1
  y : Outport  VectorParamsAs1DForOutWhenUnconnected=off
  wires:
  DataRead/1 -> y/1

== system SISO_Timer/PLC Controller Suite/__Logic/Task/Program/__Logic/XIC/RungInOverride/ForceRungInFalseRead ==
  __CoreLabelRead : Subsystem  Tag=CoreVarReadBlock  DisableCoverage=on  TreatAsAtomicUnit=on  mask{PLCBlockType=CoreLabelRead}
      mask init:
      | slplc.callbacks.initRoutineLabelRead(gcb);
      mask Help: web([docroot '/plccoder/ref/__corelabelread' '.html']);
      mask DialogControl PLCBlockTitle Prompt: Core Label Read
  Out1 : Outport  VectorParamsAs1DForOutWhenUnconnected=off
  wires:
  __CoreLabelRead/1(Out1) -> Out1/1

== system SISO_Timer/PLC Controller Suite/__Logic/Task/Program/__Logic/XIC1/BlockEnableRead/__CoreLabelRead ==
  DataRead : DataStoreRead  DataStoreName=x_PLCLabel__s4_3653__Block_Enable  IndexOptions=Index vector (dialog)  Indices=1  OutputSizes=1
  Out1 : Outport  VectorParamsAs1DForOutWhenUnconnected=off
  wires:
  DataRead/1 -> Out1/1

== system SISO_Timer/PLC Controller Suite/__Logic/Task/Program/__Logic/XIC1/Instruction_Enable/__CoreVarRead ==
  DataRead : DataStoreRead  DataStoreName=xxx_PLC_VAR_Button  IndexOptions=Index vector (dialog)  Indices=1  OutputSizes=1
  y : Outport  VectorParamsAs1DForOutWhenUnconnected=off
  wires:
  DataRead/1 -> y/1

== system SISO_Timer/PLC Controller Suite/__Logic/Task/Program/__Logic/XIC1/RungInOverride/ForceRungInFalseRead ==
  __CoreLabelRead : Subsystem  Tag=CoreVarReadBlock  DisableCoverage=on  TreatAsAtomicUnit=on  mask{PLCBlockType=CoreLabelRead}
      mask init:
      | slplc.callbacks.initRoutineLabelRead(gcb);
      mask Help: web([docroot '/plccoder/ref/__corelabelread' '.html']);
      mask DialogControl PLCBlockTitle Prompt: Core Label Read
  Out1 : Outport  VectorParamsAs1DForOutWhenUnconnected=off
  wires:
  __CoreLabelRead/1(Out1) -> Out1/1

== system SISO_Timer/PLC Controller Suite/__Logic/Task/Program/__Logic/XIC2/BlockEnableRead/__CoreLabelRead ==
  DataRead : DataStoreRead  DataStoreName=x_PLCLabel__s4_3653__Block_Enable  IndexOptions=Index vector (dialog)  Indices=1  OutputSizes=1
  Out1 : Outport  VectorParamsAs1DForOutWhenUnconnected=off
  wires:
  DataRead/1 -> Out1/1

== system SISO_Timer/PLC Controller Suite/__Logic/Task/Program/__Logic/XIC2/Instruction_Enable/__CoreVarRead ==
  DataRead : DataStoreRead  DataStoreName=xxx_PLC_VAR_St2  IndexOptions=Index vector (dialog)  Indices=1  OutputSizes=1
  y : Outport  VectorParamsAs1DForOutWhenUnconnected=off
  wires:
  DataRead/1 -> y/1

== system SISO_Timer/PLC Controller Suite/__Logic/Task/Program/__Logic/XIC2/RungInOverride/ForceRungInFalseRead ==
  __CoreLabelRead : Subsystem  Tag=CoreVarReadBlock  DisableCoverage=on  TreatAsAtomicUnit=on  mask{PLCBlockType=CoreLabelRead}
      mask init:
      | slplc.callbacks.initRoutineLabelRead(gcb);
      mask Help: web([docroot '/plccoder/ref/__corelabelread' '.html']);
      mask DialogControl PLCBlockTitle Prompt: Core Label Read
  Out1 : Outport  VectorParamsAs1DForOutWhenUnconnected=off
  wires:
  __CoreLabelRead/1(Out1) -> Out1/1

== system SISO_Timer/PLC Controller Suite/__Logic/Task/Program/__Logic/XIC3/BlockEnableRead/__CoreLabelRead ==
  DataRead : DataStoreRead  DataStoreName=x_PLCLabel__s4_3653__Block_Enable  IndexOptions=Index vector (dialog)  Indices=1  OutputSizes=1
  Out1 : Outport  VectorParamsAs1DForOutWhenUnconnected=off
  wires:
  DataRead/1 -> Out1/1

== system SISO_Timer/PLC Controller Suite/__Logic/Task/Program/__Logic/XIC3/Instruction_Enable/__CoreVarRead ==
  DataRead : DataStoreRead  DataStoreName=xxx_PLC_VAR_T  DataStoreElements=xxx_PLC_VAR_T.DN  IndexOptions=Index vector (dialog)  Indices=1  OutputSizes=1
  y : Outport  VectorParamsAs1DForOutWhenUnconnected=off
  wires:
  DataRead/1 -> y/1

== system SISO_Timer/PLC Controller Suite/__Logic/Task/Program/__Logic/XIC3/RungInOverride/ForceRungInFalseRead ==
  __CoreLabelRead : Subsystem  Tag=CoreVarReadBlock  DisableCoverage=on  TreatAsAtomicUnit=on  mask{PLCBlockType=CoreLabelRead}
      mask init:
      | slplc.callbacks.initRoutineLabelRead(gcb);
      mask Help: web([docroot '/plccoder/ref/__corelabelread' '.html']);
      mask DialogControl PLCBlockTitle Prompt: Core Label Read
  Out1 : Outport  VectorParamsAs1DForOutWhenUnconnected=off
  wires:
  __CoreLabelRead/1(Out1) -> Out1/1

== system SISO_Timer/PLC Controller Suite/__Logic/Task/Program/__Logic/XIC4/BlockEnableRead/__CoreLabelRead ==
  DataRead : DataStoreRead  DataStoreName=x_PLCLabel__s4_3653__Block_Enable  IndexOptions=Index vector (dialog)  Indices=1  OutputSizes=1
  Out1 : Outport  VectorParamsAs1DForOutWhenUnconnected=off
  wires:
  DataRead/1 -> Out1/1

== system SISO_Timer/PLC Controller Suite/__Logic/Task/Program/__Logic/XIC4/Instruction_Enable/__CoreVarRead ==
  DataRead : DataStoreRead  DataStoreName=xxx_PLC_VAR_St2  IndexOptions=Index vector (dialog)  Indices=1  OutputSizes=1
  y : Outport  VectorParamsAs1DForOutWhenUnconnected=off
  wires:
  DataRead/1 -> y/1

== system SISO_Timer/PLC Controller Suite/__Logic/Task/Program/__Logic/XIC4/RungInOverride/ForceRungInFalseRead ==
  __CoreLabelRead : Subsystem  Tag=CoreVarReadBlock  DisableCoverage=on  TreatAsAtomicUnit=on  mask{PLCBlockType=CoreLabelRead}
      mask init:
      | slplc.callbacks.initRoutineLabelRead(gcb);
      mask Help: web([docroot '/plccoder/ref/__corelabelread' '.html']);
      mask DialogControl PLCBlockTitle Prompt: Core Label Read
  Out1 : Outport  VectorParamsAs1DForOutWhenUnconnected=off
  wires:
  __CoreLabelRead/1(Out1) -> Out1/1

== system SISO_Timer/PLC Controller Suite/__Logic/Task/Program/__Logic/XIC5/BlockEnableRead/__CoreLabelRead ==
  DataRead : DataStoreRead  DataStoreName=x_PLCLabel__s4_3653__Block_Enable  IndexOptions=Index vector (dialog)  Indices=1  OutputSizes=1
  Out1 : Outport  VectorParamsAs1DForOutWhenUnconnected=off
  wires:
  DataRead/1 -> Out1/1

== system SISO_Timer/PLC Controller Suite/__Logic/Task/Program/__Logic/XIC5/Instruction_Enable/__CoreVarRead ==
  DataRead : DataStoreRead  DataStoreName=xxx_PLC_VAR_St2  IndexOptions=Index vector (dialog)  Indices=1  OutputSizes=1
  y : Outport  VectorParamsAs1DForOutWhenUnconnected=off
  wires:
  DataRead/1 -> y/1

== system SISO_Timer/PLC Controller Suite/__Logic/Task/Program/__Logic/XIC5/RungInOverride/ForceRungInFalseRead ==
  __CoreLabelRead : Subsystem  Tag=CoreVarReadBlock  DisableCoverage=on  TreatAsAtomicUnit=on  mask{PLCBlockType=CoreLabelRead}
      mask init:
      | slplc.callbacks.initRoutineLabelRead(gcb);
      mask Help: web([docroot '/plccoder/ref/__corelabelread' '.html']);
      mask DialogControl PLCBlockTitle Prompt: Core Label Read
  Out1 : Outport  VectorParamsAs1DForOutWhenUnconnected=off
  wires:
  __CoreLabelRead/1(Out1) -> Out1/1

== system SISO_Timer/PLC Controller Suite/__Logic/Task/Program/__Logic/XIO1/BlockEnableRead/__CoreLabelRead ==
  DataRead : DataStoreRead  DataStoreName=x_PLCLabel__s4_3653__Block_Enable  IndexOptions=Index vector (dialog)  Indices=1  OutputSizes=1
  Out1 : Outport  VectorParamsAs1DForOutWhenUnconnected=off
  wires:
  DataRead/1 -> Out1/1

== system SISO_Timer/PLC Controller Suite/__Logic/Task/Program/__Logic/XIO1/Instruction_Enable/__CoreVarRead ==
  DataRead : DataStoreRead  DataStoreName=xxx_PLC_VAR_St2  IndexOptions=Index vector (dialog)  Indices=1  OutputSizes=1
  y : Outport  VectorParamsAs1DForOutWhenUnconnected=off
  wires:
  DataRead/1 -> y/1
